simulink model "pwm"  (R2018a)
settings: Solver=VariableStepAuto  StartTime=0.0  StopTime=10  RelTol=1e-3
libraries: powerlib_meascontrol x3, dsparch4 x2, simulink x1
settings Model: Creator=hp  LastModifiedBy=hp

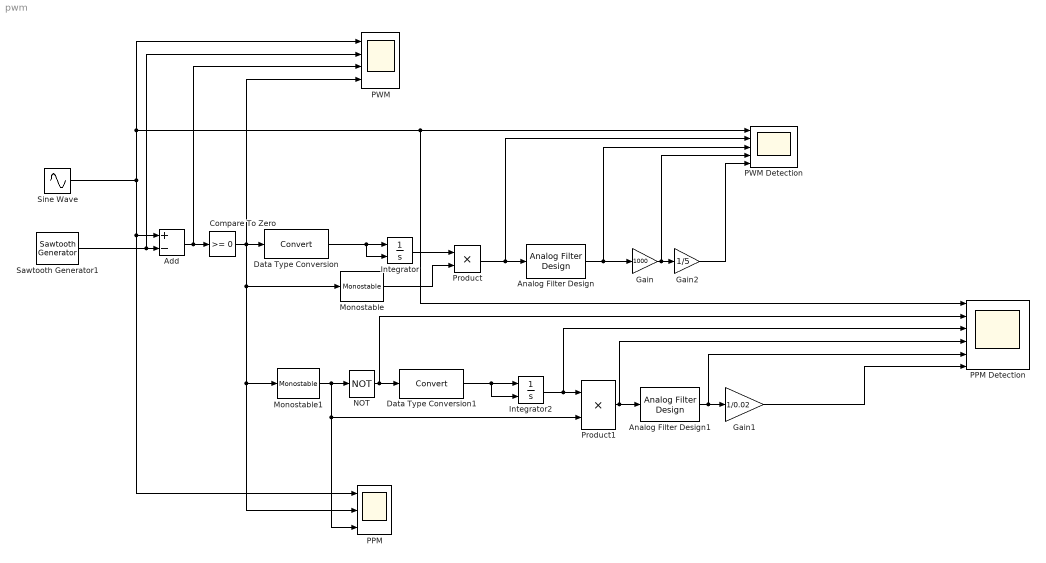
== system pwm ==
  Add : Sum  Inputs=+-
  Analog Filter Design : dsparch4/Analog Filter Design  method=Chebyshev I  filttype=Bandpass  N=4  Wlo=2*pi*0.5  Whi=2*pi*1  Rp=2  Rs=40
  Analog Filter Design1 : dsparch4/Analog Filter Design  method=Chebyshev I  filttype=Bandpass  N=8  Wlo=2*pi*0.5  Whi=2*pi*1.5  Rp=2  Rs=40
  Compare To Zero : simulink/Logic and Bit Operations/Compare To Zero  relop=>=  OutDataTypeStr=boolean
  Data Type Conversion : DataTypeConversion
  Data Type Conversion1 : DataTypeConversion
  Gain : Gain  Gain=1000
  Gain1 : Gain  Gain=1/0.02
  Gain2 : Gain  Gain=1/5
  Integrator : Integrator  ExternalReset=rising  LimitOutput=on  UpperSaturationLimit=1  LowerSaturationLimit=0
  Integrator2 : Integrator  ExternalReset=rising  LimitOutput=on  UpperSaturationLimit=1  LowerSaturationLimit=0
  Monostable : powerlib_meascontrol/Logic/Monostable  EdgeDetect=Rising  PulseDuration=0.05  ic=0  Ts=0
      settings: SourceProductName=Simscape Power Systems  SourceProductBaseCode=PS
  Monostable1 : powerlib_meascontrol/Logic/Monostable  EdgeDetect=Rising  PulseDuration=0.015  ic=0  Ts=0
      settings: SourceProductName=Simscape Power Systems  SourceProductBaseCode=PS
  NOT : Logic  Operator=NOT  IconShape=distinctive  AllPortsSameDT=off  OutDataTypeStr=boolean
  PPM : Scope  NumInputPorts=3
  PPM Detection : Scope  NumInputPorts=6
  PWM : Scope  NumInputPorts=4
  PWM Detection : Scope  NumInputPorts=5
  Product : Product
  Product1 : Product
  Sawtooth Generator1 : powerlib_meascontrol/Pulse & Signal Generators/Sawtooth Generator  Freq=15  Phase=0  Ts=0
      settings: SourceProductName=Simscape Power Systems
  Sine Wave : Sin  Frequency=2*pi*1  SampleTime=0
  wires:
  Sawtooth Generator1/1 -> PWM/2, Add/2
  Add/1 -> PWM/3, Compare To Zero/1
  Compare To Zero/1 -> PWM/4, Monostable1/1, PPM/2, Monostable/1, Data Type Conversion/1
  Data Type Conversion/1 -> Integrator/2, Integrator/1
  Integrator/1 -> Product/1
  Monostable/1 -> Product/2
  Product/1 -> PWM Detection/2, Analog Filter Design/1
  Analog Filter Design/1 -> PWM Detection/3, Gain/1
  Monostable1/1 -> PPM/3, Product1/2, NOT/1
  Integrator2/1 -> Product1/1, PPM Detection/3
  NOT/1 -> Data Type Conversion1/1, PPM Detection/2
  Product1/1 -> Analog Filter Design1/1, PPM Detection/4
  Analog Filter Design1/1 -> Gain1/1, PPM Detection/5
  Sine Wave/1 -> PPM/1, Add/1, PPM Detection/1, PWM Detection/1, PWM/1
  Gain/1 -> PWM Detection/4, Gain2/1
  Gain2/1 -> PWM Detection/5
  Data Type Conversion1/1 -> Integrator2/1, Integrator2/2
  Gain1/1 -> PPM Detection/6
